simulink model "p5p3d"  (Simulink 9.0)
settings: Solver=ode45  StartTime=0.0  StopTime=simtime  RelTol=1e-3  EnableMultiTasking=on
values from neighbouring files (symbols this model uses):
  ref = 30    [p5p3b_init.m]    (also in p5p3c_init.m; p5p3d_init.m)
libraries: simulink x2, cstblocks x1
settings Model: Creator=markh  LastModifiedBy=bruker
settings DataIOCC: LimitDataPoints=on  SignalLoggingSaveFormat=ModelDataLogs  SignalLoggingName=sigsOut
settings OptimizationCC: InitFltsAndDblsToZero=on
settings DebuggingCC: SaveWithParameterizedLinksMsg=none  SignalResolutionControl=TryResolveAllWithWarning  MultiTaskDSMMsg=warning  MultiTaskCondExecSysMsg=none  FcnCallInpInsideContextMsg=warning  StateNameClashWarn=warning  StrictBusMsg=None
settings HardwareCC: TargetUnknown=on
settings GRTTargetCC: TargetFcnLib=ansi_tfl_tmw.mat  GeneratePreprocessorConditionals=Disable all  CombineOutputUpdateFcns=off  GRTInterface=on

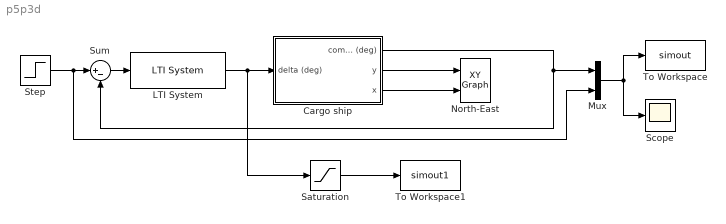
== system p5p3d ==
  Cargo ship : Subsystem  mask(Simple shipmodel for a cargo ship){noise=on, current=off, logic=on}
      mask prompts: noise "measurement noise"; logic "waves"
      mask help:
      | Measurement noise:
      | 	checked = noise on
      | 	unchecked = noise off
      |
      | Current:
      | 	checked = current on
      | 	unchecked = current off
      |
      | Waves:
      | 	checked = waves on
      | 	unchecked = waves off
      |
      | Author: Jørgen Spjøtvold, 9/10-2003
      | TTK 4115 Linear system theory.
      | Modified by Jostein Bakkeheim 26/10-2006
  LTI System : cstblocks/LTI System  sys=reg_sys  IC=[]
  Mux : Mux  Inputs=2
  North-East : simulink/Sinks/XY Graph  xmin=-5000  xmax=5000  ymin=-5000  ymax=5000  st=-1
  Saturation : Saturate  UpperLimit=45  LowerLimit=-45
  Scope : Scope
  Step : Step  Time=0  After=ref  SampleTime=0
  Sum : Sum  Inputs=|+-
  To Workspace : ToWorkspace  VariableName=simout  SaveFormat=Timeseries  SampleTime=-1
  To Workspace1 : ToWorkspace  VariableName=simout1  SaveFormat=Timeseries  SampleTime=-1
  wires:
  Cargo ship/3(x) -> North-East/2
  Cargo ship/2(y) -> North-East/1
  Cargo ship/1(compass (deg)) -> Mux/1, Sum/2
  LTI System/1 -> Saturation/1, Cargo ship/1(delta (deg))
  Step/1 -> Mux/2, Sum/1
  Sum/1 -> LTI System/1
  Mux/1 -> Scope/1, To Workspace/1
  Saturation/1 -> To Workspace1/1

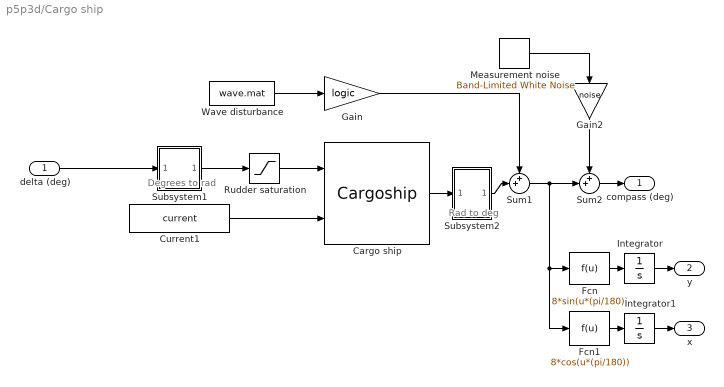
== system p5p3d/Cargo ship ==
  note: Degrees to rad
  note: Rad to deg
  delta (deg) : Inport
  Cargo ship : S-Function  FunctionName=Cargoship  SFunctionDeploymentMode=off  EnableBusSupport=off  mask(Cargo ship){}
      mask help:
      | S-function which simulates a cargo ship.
      |
      | Author: Jørgen Spjøtvold
      | 20.10-2003
      | Modified by Jostein Bakkeheim 27.10.2006
  Current1 : Constant  Value=current
  Fcn : Fcn  Expr=8*sin(u*(pi/180))
  Fcn1 : Fcn  Expr=8*cos(u*(pi/180))
  Gain : Gain  Gain=logic  SaturateOnIntegerOverflow=on  OutDataTypeStr=Inherit: Same as input  ParamDataTypeStr=Inherit: Same as input
  Gain2 : Gain  Gain=noise  SaturateOnIntegerOverflow=on  OutDataTypeStr=Inherit: Same as input  ParamDataTypeStr=Inherit: Same as input
  Integrator : Integrator
  Integrator1 : Integrator
  Measurement noise : simulink/Sources/Band-Limited White Noise  Cov=[0.001]  Ts=.5  seed=[23341]
  Rudder saturation : Saturate  UpperLimit=45*(pi/180)  LowerLimit=-45*(pi/180)
  Subsystem1 : Subsystem  mask(degrees to radians){}
      mask help: Converts degrees to radians
      mask Display: fprintf('D2R');
  Subsystem2 : Subsystem  mask(radians to degrees){}
      mask help: Converts radians to degrees
      mask Display: fprintf('R2D');
  Sum1 : Sum  Inputs=++|  SaturateOnIntegerOverflow=on
  Sum2 : Sum  Inputs=++|  SaturateOnIntegerOverflow=on
  Wave disturbance : FromFile  FileName=wave.mat  SampleTime=0
  compass (deg) : Outport
  y : Outport  Port=2
  x : Outport  Port=3
  wires:
  delta (deg)/1 -> Subsystem1/1(In1)
  Fcn/1 -> Integrator/1
  Integrator/1 -> y/1
  Fcn1/1 -> Integrator1/1
  Integrator1/1 -> x/1
  Wave disturbance/1 -> Gain/1
  Subsystem2/1(Out1) -> Sum1/2
  Gain/1 -> Sum1/1
  Sum1/1 -> Fcn/1, Fcn1/1, Sum2/2
  Cargo ship/1 -> Subsystem2/1(In1)
  Subsystem1/1(Out1) -> Rudder saturation/1
  Rudder saturation/1 -> Cargo ship/1
  Sum2/1 -> compass (deg)/1
  Measurement noise/1 -> Gain2/1
  Gain2/1 -> Sum2/1
  Current1/1 -> Cargo ship/2

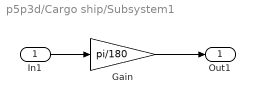
== system p5p3d/Cargo ship/Subsystem1 ==
  In1 : Inport
  Gain : Gain  Gain=pi/180  SaturateOnIntegerOverflow=on  OutDataTypeStr=Inherit: Same as input  ParamDataTypeStr=Inherit: Same as input
  Out1 : Outport
  wires:
  Gain/1 -> Out1/1
  In1/1 -> Gain/1

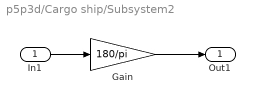
== system p5p3d/Cargo ship/Subsystem2 ==
  In1 : Inport
  Gain : Gain  Gain=180/pi  SaturateOnIntegerOverflow=on  OutDataTypeStr=Inherit: Same as input  ParamDataTypeStr=Inherit: Same as input
  Out1 : Outport
  wires:
  Gain/1 -> Out1/1
  In1/1 -> Gain/1
